simulink model "system3"  (R2019a)
settings: Solver=ode4  StartTime=0.0  StopTime=50  FixedStep=0.001  RelTol=1e-3
settings Model: Creator=vmali  LastModifiedBy=vmali

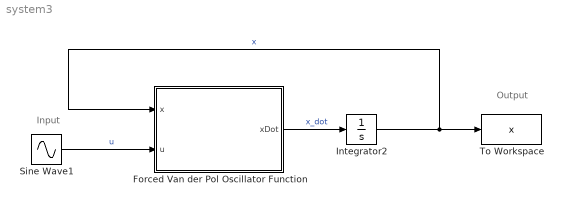
== system system3 ==
  note: Output
  note: Input
  Forced Van der Pol Oscillator Function : MATLAB Function  TreatAsAtomicUnit=on
  Integrator2 : Integrator
  Sine Wave1 : Sin  Amplitude=1.2  Frequency=0.2*pi  SampleTime=0
      settings: AttributesFormatString=|
      | Amplitude = %<Amplitude>,
      | Frequency = %<Frequency>
  To Workspace : ToWorkspace  VariableName=x  SaveFormat=Structure With Time  SampleTime=-1
      settings: AttributesFormatString=%<Name>
  wires:
  Sine Wave1/1 -> Forced Van der Pol Oscillator Function/2(u)  "u"
  Forced Van der Pol Oscillator Function/1(xDot) -> Integrator2/1  "x_dot"
  Integrator2/1 -> To Workspace/1, Forced Van der Pol Oscillator Function/1(x)  "x"

== matlab function system3/Forced Van der Pol Oscillator Function ==
  data: x input; u input; xDot output
function xDot = f(x,u)
% Function f of x' = f(x,u,t)
% x == states
% u == inputs
% t == time
% p == parameters

%Give the input parameters

mu = 8.53;

% grab memory
xDot = zeros(2,1);

% fill in f of x' = f(x,u,t)
xDot(1) = x(2);
xDot(2) = mu*(1-x(1)^2)*x(2) - x(1) + u;
